simulink model "UART_Overview"  (R2014b)
settings: Solver=ode45  StartTime=0.0  StopTime=10.0  RelTol=1e-3
libraries: instrumentlib x2
settings Model: Creator=Ben Windo  LastModifiedBy=Ben Windo

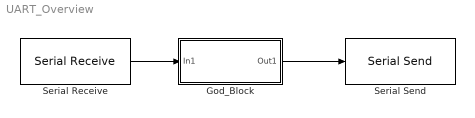
== system UART_Overview ==
  God_Block : Subsystem
  Serial Receive : instrumentlib/Serial Receive  ComPortMenu=<Please select a port...>  ComPort=<Please select a port...>  Terminator=<none>  DataSize=[1 1]  DataType=uint8  EnableBlockingMode=on  ActionDataUnavailable=Output last received value  CustomValue=0  SampleTime=0.01
  Serial Send : instrumentlib/Serial Send  ComPortMenu=<Please select a port...>  ComPort=<Please select a port...>  Terminator=<none>  EnableBlockingMode=on
  wires:
  God_Block/1(Out1) -> Serial Send/1
  Serial Receive/1 -> God_Block/1(In1)

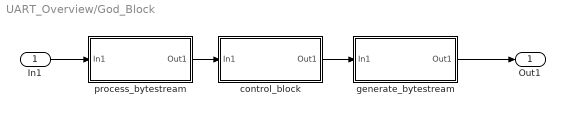
== system UART_Overview/God_Block ==
  In1 : Inport
  "control_block " : Subsystem
  generate_bytestream : Subsystem
  "process_bytestream " : Subsystem
  Out1 : Outport
  wires:
  "process_bytestream "/1(Out1) -> "control_block "/1(In1)
  "control_block "/1(Out1) -> generate_bytestream/1(In1)
  generate_bytestream/1(Out1) -> Out1/1
  In1/1 -> "process_bytestream "/1(In1)

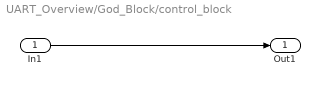
== system UART_Overview/God_Block/control_block  ==
  In1 : Inport
  Out1 : Outport
  wires:
  In1/1 -> Out1/1

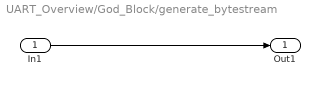
== system UART_Overview/God_Block/generate_bytestream ==
  In1 : Inport
  Out1 : Outport
  wires:
  In1/1 -> Out1/1

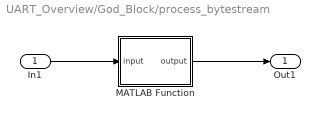
== system UART_Overview/God_Block/process_bytestream  ==
  In1 : Inport
  MATLAB Function : MATLAB Function  TreatAsAtomicUnit=on
  Out1 : Outport
  wires:
  In1/1 -> MATLAB Function/1(input)
  MATLAB Function/1(output) -> Out1/1

== matlab function UART_Overview/God_Block/process_bytestream /MATLAB Function ==
  data: input input; output output

function output = process_bytestream(input)
verify_checksum(input);
end
function output = verify_checksum(input)

sum1=0;
sum2=0;
for i = 1:3
 sum1 = mod((sum1 + input(i)), 255);
 input(i);
 sum2 = mod((sum2 + sum1), 255);
end

fletcher = typecast([sum1,sum2],'uint16');
checksum = typecast([input(4), input(5)], 'uint16');
output = (checksum == fletcher);
%output = [checksum, fletcher];
end
